simulink model "atrias_system"  (R2015a)
settings: Solver=FixedStepDiscrete  StartTime=0.0  StopTime=inf  FixedStep=sample_time  RelTol=1e-3
undefined symbols (not defined in the file or in its folder): gui_disable_cmd, gui_enable_cmd, gui_estop_cmd, gui_reset_cmd, HIP_CURRENT_LIMIT, HIP_MOTOR_CONSTANT, HIP_MTR_GEAR_RATIO, HIP_MTR_MAX_TORQUE, LEFT_MOTOR_HIP_DIRECTION, LEG1_MOTOR_A_DIRECTION, LEG1_MOTOR_B_DIRECTION, LEG2_MOTOR_A_DIRECTION, LEG2_MOTOR_B_DIRECTION, LEG_CURRENT_LIMIT, LEG_MOTOR_CONSTANT, LEG_MTR_GEAR_RATIO, LEG_MTR_MAX_TORQUE, MEDULLA_ADC_MAX_VOLTS, MEDULLA_ADC_OFFSET_COUNTS, MEDULLA_STATE_ERROR, MEDULLA_STATE_HALT, MEDULLA_STATE_IDLE, MEDULLA_STATE_RESET, MEDULLA_STATE_RUN, MOTOR_POSITION_LIMITS_LOWER, MOTOR_POSITION_LIMITS_UPPER, MTR_HIP_MAX_CURRENT, MTR_MAX_CONT_CURRENT, MTR_MAX_COUNT, MTR_MAX_CURRENT, RIGHT_MOTOR_HIP_DIRECTION
libraries: xpcethercatlib x188, simulink x36, slrtlib x2
(part 3 of 3)

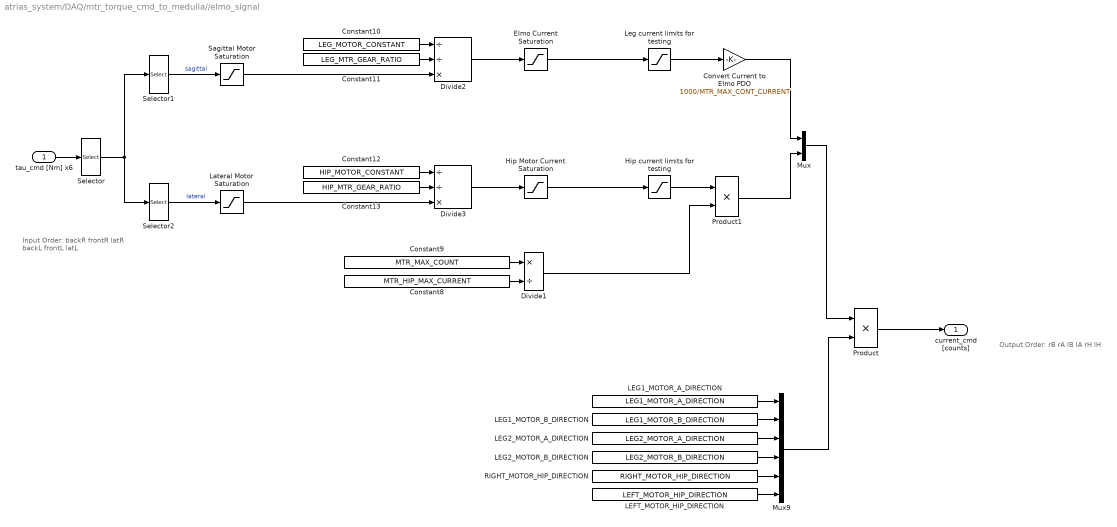
== system atrias_system/DAQ/mtr_torque_cmd_to_medulla//elmo_signal ==
  note: Output Order:
      | rB
      | rA
      | lB
      | lA
      | rH
      | lH
  note: Input Order:
      |
      | backR
      | frontR
      | latR
      | backL
      | frontL
      | latL
  tau_cmd [Nm] x6 : Inport
  Constant10 : Constant  Value=LEG_MOTOR_CONSTANT
  Constant11 : Constant  Value=LEG_MTR_GEAR_RATIO
  Constant12 : Constant  Value=HIP_MOTOR_CONSTANT
  Constant13 : Constant  Value=HIP_MTR_GEAR_RATIO
  Constant8 : Constant  Value=MTR_HIP_MAX_CURRENT
  Constant9 : Constant  Value=MTR_MAX_COUNT
  Convert Current to Elmo PDO : Gain  Gain=1000/MTR_MAX_CONT_CURRENT
  Divide1 : Product  Inputs=*/
  Divide2 : Product  Inputs=//*
  Divide3 : Product  Inputs=//*
  Elmo Current Saturation : Saturate  UpperLimit=MTR_MAX_CURRENT  LowerLimit=-MTR_MAX_CURRENT
      settings: AttributesFormatString=Top: %<UpperLimit>\nBottom: %<LowerLimit>
  Hip Motor Current Saturation : Saturate  UpperLimit=MTR_HIP_MAX_CURRENT  LowerLimit=-MTR_HIP_MAX_CURRENT
      settings: AttributesFormatString=Top: %<UpperLimit>\nBottom: %<LowerLimit>
  Hip current limits for testing : Saturate  UpperLimit=HIP_CURRENT_LIMIT  LowerLimit=-HIP_CURRENT_LIMIT
      settings: AttributesFormatString=Top: %<UpperLimit>\nBottom: %<LowerLimit>
  LEFT_MOTOR_HIP_DIRECTION : Constant  Value=LEFT_MOTOR_HIP_DIRECTION
  LEG1_MOTOR_A_DIRECTION : Constant  Value=LEG1_MOTOR_A_DIRECTION
  LEG1_MOTOR_B_DIRECTION : Constant  Value=LEG1_MOTOR_B_DIRECTION
  LEG2_MOTOR_A_DIRECTION : Constant  Value=LEG2_MOTOR_A_DIRECTION
  LEG2_MOTOR_B_DIRECTION : Constant  Value=LEG2_MOTOR_B_DIRECTION
  Lateral Motor Saturation : Saturate  UpperLimit=HIP_MTR_MAX_TORQUE  LowerLimit=-HIP_MTR_MAX_TORQUE
      settings: AttributesFormatString=Top: %<UpperLimit>\nBottom: %<LowerLimit>
  Leg current limits for testing : Saturate  UpperLimit=LEG_CURRENT_LIMIT  LowerLimit=-LEG_CURRENT_LIMIT
      settings: AttributesFormatString=Top: %<UpperLimit>\nBottom: %<LowerLimit>
  Mux : Mux  Inputs=2
  Mux9 : Mux  Inputs=6
  Product : Product  RndMeth=Zero
  Product1 : Product  RndMeth=Zero
  RIGHT_MOTOR_HIP_DIRECTION : Constant  Value=RIGHT_MOTOR_HIP_DIRECTION
  Sagittal Motor Saturation : Saturate  UpperLimit=LEG_MTR_MAX_TORQUE  LowerLimit=-LEG_MTR_MAX_TORQUE
      settings: AttributesFormatString=Top: %<UpperLimit>\nBottom: %<LowerLimit>
  Selector : Selector  InputPortWidth=6  Indices=[1 2 4 5 3 6]
  Selector1 : Selector  InputPortWidth=6  Indices=[1 2 3 4]
  Selector2 : Selector  InputPortWidth=6  Indices=[5 6]
  current_cmd [counts] : Outport
  wires:
  Lateral Motor Saturation/1 -> Divide3/3
  Sagittal Motor Saturation/1 -> Divide2/3
  Convert Current to Elmo PDO/1 -> Mux/1
  Mux/1 -> Product/1
  Divide2/1 -> Elmo Current Saturation/1
  Constant12/1 -> Divide3/1
  Constant13/1 -> Divide3/2
  Constant10/1 -> Divide2/1
  Constant11/1 -> Divide2/2
  Selector2/1 -> Lateral Motor Saturation/1  "lateral"
  Selector1/1 -> Sagittal Motor Saturation/1  "sagittal"
  LEG1_MOTOR_A_DIRECTION/1 -> Mux9/1
  LEG1_MOTOR_B_DIRECTION/1 -> Mux9/2
  LEG2_MOTOR_A_DIRECTION/1 -> Mux9/3
  Mux9/1 -> Product/2
  LEG2_MOTOR_B_DIRECTION/1 -> Mux9/4
  RIGHT_MOTOR_HIP_DIRECTION/1 -> Mux9/5
  LEFT_MOTOR_HIP_DIRECTION/1 -> Mux9/6
  Product/1 -> current_cmd [counts]/1
  tau_cmd [Nm] x6/1 -> Selector/1
  Selector/1 -> Selector1/1, Selector2/1
  Hip Motor Current Saturation/1 -> Hip current limits for testing/1
  Divide3/1 -> Hip Motor Current Saturation/1
  Constant9/1 -> Divide1/1
  Constant8/1 -> Divide1/2
  Divide1/1 -> Product1/2
  Elmo Current Saturation/1 -> Leg current limits for testing/1
  Product1/1 -> Mux/2
  Hip current limits for testing/1 -> Product1/1
  Leg current limits for testing/1 -> Convert Current to Elmo PDO/1

== system atrias_system/Start Controller/Hold Start Time ==
  Time In : Inport  OutDataTypeStr=double
  Enable : EnablePort
  Time Out : Outport  OutDataTypeStr=double
  wires:
  Time In/1 -> Time Out/1

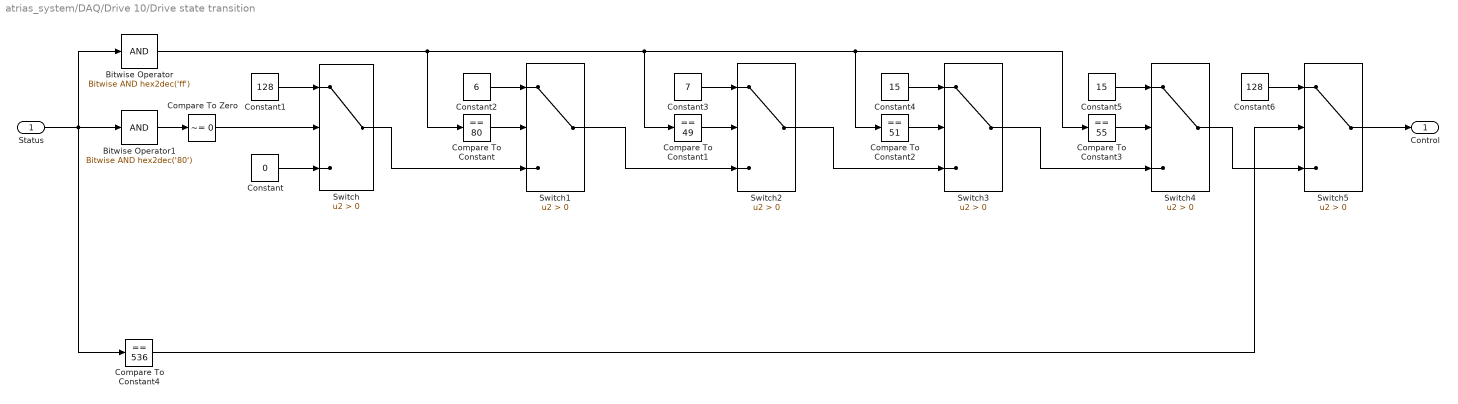
== system atrias_system/DAQ/Drive 10/Drive state transition ==
  Status : Inport
  Bitwise Operator : simulink/Logic and Bit Operations/Bitwise Operator  logicop=AND  UseBitMask=on  BitMask=hex2dec('ff')  BitMaskRealWorld=Stored Integer
  Bitwise Operator1 : simulink/Logic and Bit Operations/Bitwise Operator  logicop=AND  UseBitMask=on  BitMask=hex2dec('80')  BitMaskRealWorld=Stored Integer
  Compare To Constant : simulink/Logic and Bit Operations/Compare To Constant  relop===  const=80  OutDataTypeStr=boolean
  Compare To Constant1 : simulink/Logic and Bit Operations/Compare To Constant  relop===  const=49  OutDataTypeStr=boolean
  Compare To Constant2 : simulink/Logic and Bit Operations/Compare To Constant  relop===  const=51  OutDataTypeStr=boolean
  Compare To Constant3 : simulink/Logic and Bit Operations/Compare To Constant  relop===  const=55  OutDataTypeStr=boolean
  Compare To Constant4 : simulink/Logic and Bit Operations/Compare To Constant  relop===  const=536  OutDataTypeStr=boolean
  Compare To Zero : simulink/Logic and Bit Operations/Compare To Zero  relop=~=  OutDataTypeStr=boolean
  Constant : Constant  Value=0  OutDataTypeStr=uint16
  Constant1 : Constant  Value=128  OutDataTypeStr=uint16
  Constant2 : Constant  Value=6  OutDataTypeStr=uint16
  Constant3 : Constant  Value=7  OutDataTypeStr=uint16
  Constant4 : Constant  Value=15  OutDataTypeStr=uint16
  Constant5 : Constant  Value=15  OutDataTypeStr=uint16
  Constant6 : Constant  Value=128  OutDataTypeStr=uint16
  Switch{,1..5} (6 alike) : Switch  Criteria=u2 > Threshold
  Control : Outport
  wires:
  Constant6/1 -> Switch5/1
  Switch5/1 -> Control/1
  Compare To Constant4/1 -> Switch5/2
  Switch4/1 -> Switch5/3
  Constant5/1 -> Switch4/1
  Switch3/1 -> Switch4/3
  Compare To Constant3/1 -> Switch4/2
  Constant4/1 -> Switch3/1
  Switch2/1 -> Switch3/3
  Compare To Constant2/1 -> Switch3/2
  Constant3/1 -> Switch2/1
  Switch1/1 -> Switch2/3
  Compare To Constant1/1 -> Switch2/2
  Constant2/1 -> Switch1/1
  Bitwise Operator/1 -> Compare To Constant/1, Compare To Constant1/1, Compare To Constant2/1, Compare To Constant3/1
  Switch/1 -> Switch1/3
  Compare To Constant/1 -> Switch1/2
  Constant/1 -> Switch/3
  Constant1/1 -> Switch/1
  Compare To Zero/1 -> Switch/2
  Bitwise Operator1/1 -> Compare To Zero/1
  Status/1 -> Bitwise Operator1/1, Bitwise Operator/1, Compare To Constant4/1

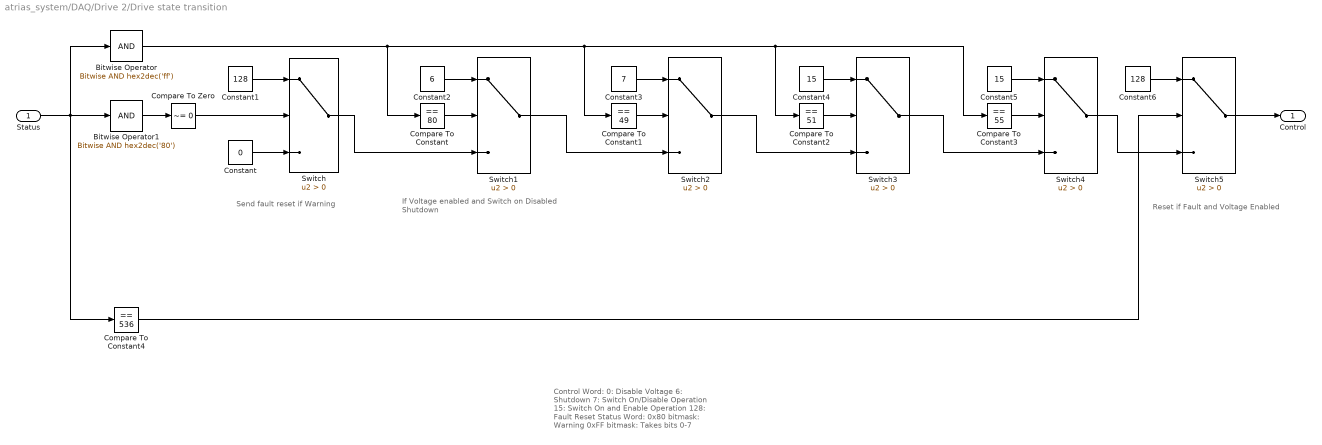
== system atrias_system/DAQ/Drive 2/Drive state transition ==
  note: If Voltage enabled and Switch on Disabled
      | Shutdown
  note: Reset if Fault and Voltage Enabled
  note: Send fault reset if Warning
  note: Control Word:
      | 0: Disable Voltage
      | 6: Shutdown
      | 7: Switch On/Disable Operation
      | 15: Switch On and Enable Operation
      | 128: Fault Reset
      |
      | Status Word:
      | 0x80 bitmask: Warning
      | 0xFF bitmask: Takes bits 0-7
  Status : Inport
  Bitwise Operator : simulink/Logic and Bit Operations/Bitwise Operator  logicop=AND  UseBitMask=on  BitMask=hex2dec('ff')  BitMaskRealWorld=Stored Integer
  Bitwise Operator1 : simulink/Logic and Bit Operations/Bitwise Operator  logicop=AND  UseBitMask=on  BitMask=hex2dec('80')  BitMaskRealWorld=Stored Integer
  Compare To Constant : simulink/Logic and Bit Operations/Compare To Constant  relop===  const=80  OutDataTypeStr=boolean
  Compare To Constant1 : simulink/Logic and Bit Operations/Compare To Constant  relop===  const=49  OutDataTypeStr=boolean
  Compare To Constant2 : simulink/Logic and Bit Operations/Compare To Constant  relop===  const=51  OutDataTypeStr=boolean
  Compare To Constant3 : simulink/Logic and Bit Operations/Compare To Constant  relop===  const=55  OutDataTypeStr=boolean
  Compare To Constant4 : simulink/Logic and Bit Operations/Compare To Constant  relop===  const=536  OutDataTypeStr=boolean
  Compare To Zero : simulink/Logic and Bit Operations/Compare To Zero  relop=~=  OutDataTypeStr=boolean
  Constant : Constant  Value=0  OutDataTypeStr=uint16
  Constant1 : Constant  Value=128  OutDataTypeStr=uint16
  Constant2 : Constant  Value=6  OutDataTypeStr=uint16
  Constant3 : Constant  Value=7  OutDataTypeStr=uint16
  Constant4 : Constant  Value=15  OutDataTypeStr=uint16
  Constant5 : Constant  Value=15  OutDataTypeStr=uint16
  Constant6 : Constant  Value=128  OutDataTypeStr=uint16
  Switch{,1..5} (6 alike) : Switch  Criteria=u2 > Threshold
  Control : Outport
  wires:
  Status/1 -> Compare To Constant4/1, Bitwise Operator/1, Bitwise Operator1/1
  Bitwise Operator1/1 -> Compare To Zero/1
  Compare To Zero/1 -> Switch/2
  Constant1/1 -> Switch/1
  Constant/1 -> Switch/3
  Compare To Constant/1 -> Switch1/2
  Switch/1 -> Switch1/3
  Bitwise Operator/1 -> Compare To Constant3/1, Compare To Constant2/1, Compare To Constant1/1, Compare To Constant/1
  Constant2/1 -> Switch1/1
  Compare To Constant1/1 -> Switch2/2
  Switch1/1 -> Switch2/3
  Constant3/1 -> Switch2/1
  Compare To Constant2/1 -> Switch3/2
  Switch2/1 -> Switch3/3
  Constant4/1 -> Switch3/1
  Compare To Constant3/1 -> Switch4/2
  Switch3/1 -> Switch4/3
  Constant5/1 -> Switch4/1
  Switch4/1 -> Switch5/3
  Compare To Constant4/1 -> Switch5/2
  Switch5/1 -> Control/1
  Constant6/1 -> Switch5/1

== system atrias_system/DAQ/Drive 3/Drive state transition ==
  Status : Inport
  Bitwise Operator : simulink/Logic and Bit Operations/Bitwise Operator  logicop=AND  UseBitMask=on  BitMask=hex2dec('ff')  BitMaskRealWorld=Stored Integer
  Bitwise Operator1 : simulink/Logic and Bit Operations/Bitwise Operator  logicop=AND  UseBitMask=on  BitMask=hex2dec('80')  BitMaskRealWorld=Stored Integer
  Compare To Constant : simulink/Logic and Bit Operations/Compare To Constant  relop===  const=80  OutDataTypeStr=boolean
  Compare To Constant1 : simulink/Logic and Bit Operations/Compare To Constant  relop===  const=49  OutDataTypeStr=boolean
  Compare To Constant2 : simulink/Logic and Bit Operations/Compare To Constant  relop===  const=51  OutDataTypeStr=boolean
  Compare To Constant3 : simulink/Logic and Bit Operations/Compare To Constant  relop===  const=55  OutDataTypeStr=boolean
  Compare To Constant4 : simulink/Logic and Bit Operations/Compare To Constant  relop===  const=536  OutDataTypeStr=boolean
  Compare To Zero : simulink/Logic and Bit Operations/Compare To Zero  relop=~=  OutDataTypeStr=boolean
  Constant : Constant  Value=0  OutDataTypeStr=uint16
  Constant1 : Constant  Value=128  OutDataTypeStr=uint16
  Constant2 : Constant  Value=6  OutDataTypeStr=uint16
  Constant3 : Constant  Value=7  OutDataTypeStr=uint16
  Constant4 : Constant  Value=15  OutDataTypeStr=uint16
  Constant5 : Constant  Value=15  OutDataTypeStr=uint16
  Constant6 : Constant  Value=128  OutDataTypeStr=uint16
  Switch{,1..5} (6 alike) : Switch  Criteria=u2 > Threshold
  Control : Outport
  wires:
  Status/1 -> Compare To Constant4/1, Bitwise Operator/1, Bitwise Operator1/1
  Bitwise Operator1/1 -> Compare To Zero/1
  Compare To Zero/1 -> Switch/2
  Constant1/1 -> Switch/1
  Constant/1 -> Switch/3
  Compare To Constant/1 -> Switch1/2
  Switch/1 -> Switch1/3
  Bitwise Operator/1 -> Compare To Constant3/1, Compare To Constant2/1, Compare To Constant1/1, Compare To Constant/1
  Constant2/1 -> Switch1/1
  Compare To Constant1/1 -> Switch2/2
  Switch1/1 -> Switch2/3
  Constant3/1 -> Switch2/1
  Compare To Constant2/1 -> Switch3/2
  Switch2/1 -> Switch3/3
  Constant4/1 -> Switch3/1
  Compare To Constant3/1 -> Switch4/2
  Switch3/1 -> Switch4/3
  Constant5/1 -> Switch4/1
  Switch4/1 -> Switch5/3
  Compare To Constant4/1 -> Switch5/2
  Switch5/1 -> Control/1
  Constant6/1 -> Switch5/1

== system atrias_system/DAQ/Drive 9/Drive state transition ==
  Status : Inport
  Bitwise Operator : simulink/Logic and Bit Operations/Bitwise Operator  logicop=AND  UseBitMask=on  BitMask=hex2dec('ff')  BitMaskRealWorld=Stored Integer
  Bitwise Operator1 : simulink/Logic and Bit Operations/Bitwise Operator  logicop=AND  UseBitMask=on  BitMask=hex2dec('80')  BitMaskRealWorld=Stored Integer
  Compare To Constant : simulink/Logic and Bit Operations/Compare To Constant  relop===  const=80  OutDataTypeStr=boolean
  Compare To Constant1 : simulink/Logic and Bit Operations/Compare To Constant  relop===  const=49  OutDataTypeStr=boolean
  Compare To Constant2 : simulink/Logic and Bit Operations/Compare To Constant  relop===  const=51  OutDataTypeStr=boolean
  Compare To Constant3 : simulink/Logic and Bit Operations/Compare To Constant  relop===  const=55  OutDataTypeStr=boolean
  Compare To Constant4 : simulink/Logic and Bit Operations/Compare To Constant  relop===  const=536  OutDataTypeStr=boolean
  Compare To Zero : simulink/Logic and Bit Operations/Compare To Zero  relop=~=  OutDataTypeStr=boolean
  Constant : Constant  Value=0  OutDataTypeStr=uint16
  Constant1 : Constant  Value=128  OutDataTypeStr=uint16
  Constant2 : Constant  Value=6  OutDataTypeStr=uint16
  Constant3 : Constant  Value=7  OutDataTypeStr=uint16
  Constant4 : Constant  Value=15  OutDataTypeStr=uint16
  Constant5 : Constant  Value=15  OutDataTypeStr=uint16
  Constant6 : Constant  Value=128  OutDataTypeStr=uint16
  Switch{,1..5} (6 alike) : Switch  Criteria=u2 > Threshold
  Control : Outport
  wires:
  Status/1 -> Compare To Constant4/1, Bitwise Operator/1, Bitwise Operator1/1
  Bitwise Operator1/1 -> Compare To Zero/1
  Compare To Zero/1 -> Switch/2
  Constant1/1 -> Switch/1
  Constant/1 -> Switch/3
  Compare To Constant/1 -> Switch1/2
  Switch/1 -> Switch1/3
  Bitwise Operator/1 -> Compare To Constant3/1, Compare To Constant2/1, Compare To Constant1/1, Compare To Constant/1
  Constant2/1 -> Switch1/1
  Compare To Constant1/1 -> Switch2/2
  Switch1/1 -> Switch2/3
  Constant3/1 -> Switch2/1
  Compare To Constant2/1 -> Switch3/2
  Switch2/1 -> Switch3/3
  Constant4/1 -> Switch3/1
  Compare To Constant3/1 -> Switch4/2
  Switch3/1 -> Switch4/3
  Constant5/1 -> Switch4/1
  Switch4/1 -> Switch5/3
  Compare To Constant4/1 -> Switch5/2
  Switch5/1 -> Control/1
  Constant6/1 -> Switch5/1

== matlab function atrias_system/DAQ/logic_voltage_volts ==
  data: u input; volt output; MEDULLA_ADC_OFFSET_COUNTS parameter; MEDULLA_ADC_MAX_VOLTS parameter
function volt = fcn(u, MEDULLA_ADC_OFFSET_COUNTS, MEDULLA_ADC_MAX_VOLTS)
% Taken from Medulla.cpp in the ATRIAS medulla drivers
% at code.google.com/p/atrias
adcReadingVolts = (u - MEDULLA_ADC_OFFSET_COUNTS) * MEDULLA_ADC_MAX_VOLTS/4095;
volt            = 6 * adcReadingVolts;

== matlab function atrias_system/DAQ/medulla_errors ==
  data: u input; errors output
function errors = fcn(u)
% right back, right front, left back, left front, left lateral, right lateral, boom
errors = reshape(bsxfun(@bitand,u,2.^[0 1 2 3 4 5 6 7]),[],1);

== matlab function atrias_system/Compute State Command ==
  data: medulla_states input uint8; elmo_enable output; medulla_cmd output; should_estop input boolean; should_halt input boolean; gui_enable_cmd parameter boolean; gui_disable_cmd parameter boolean; gui_reset_cmd parameter boolean; gui_estop_cmd parameter boolean; MEDULLA_STATE_IDLE parameter uint8; MEDULLA_STATE_RUN parameter uint8; MEDULLA_STATE_HALT parameter uint8; MEDULLA_STATE_ERROR parameter uint8; MEDULLA_STATE_RESET parameter uint8; any_halt output boolean
function [elmo_enable,medulla_cmd,any_halt] = fcn(medulla_states,      ...
                                                  should_estop,        ...
                                                  should_halt,         ...
                                                  gui_enable_cmd,      ...
                                                  gui_disable_cmd,     ...
                                                  gui_reset_cmd,       ...
                                                  gui_estop_cmd,       ...
                                                  MEDULLA_STATE_IDLE,  ...
                                                  MEDULLA_STATE_RUN,   ...
                                                  MEDULLA_STATE_HALT,  ...
                                                  MEDULLA_STATE_ERROR, ...
                                                  MEDULLA_STATE_RESET)
%#codegen

% Count the number of medullas in each state
any_idle  = any(medulla_states == MEDULLA_STATE_IDLE );
any_reset = any(medulla_states == MEDULLA_STATE_RESET);
any_run   = any(medulla_states == MEDULLA_STATE_RUN  );
any_halt  = any(medulla_states == MEDULLA_STATE_HALT );
any_estop = any(medulla_states == MEDULLA_STATE_ERROR);

% The GUI estop command should do the same thing as asserting the
% should_estop line
should_estop = should_estop || gui_estop_cmd;

% Compute whether or not to reset based on the current states and the
% GUI's input
should_reset = gui_reset_cmd  && ...
              ~gui_enable_cmd && ... % Make sure we're not about to re-enable (precaution)
               any_estop      && ... % A medulla must be e-stopped (precaution)
              ~any_halt       && ... % No medullas may be halting (precaution)
              ~any_run;              % No medullas may be running (precaution)

% Send an E-Stop first if the safeties are engaging, so this can't fail.
% Also send an E-Stop if any medullas are E-stopped, unless the GUI is
% sending a reset command
if ((any_run || any_halt) && should_estop) || (any_estop && ~should_reset)
    elmo_enable = false;
    medulla_cmd = MEDULLA_STATE_ERROR;
    return
end

% If any Medullas are halting, automatically command halt for all.
% If we want to command a halt while we're in run, command a halt.
if any_halt || (any_run && should_halt)
    elmo_enable = true;
    medulla_cmd = MEDULLA_STATE_HALT;
    return
end

% Allow for GUI-commanded resets. Make sure an enable command isn't being
% sent as an enable precaution
if should_reset || any_reset
    elmo_enable = false;
    medulla_cmd = MEDULLA_STATE_RESET;
    return
end

% Past this point, the robot should be either enabled or disabled
% (no E-Stops or halts)

% Allow the GUI to disable the robot.
% For now, there is no soft shutdown.
if gui_disable_cmd
    elmo_enable = false;
    medulla_cmd = MEDULLA_STATE_IDLE;
    return
end

% Allow for enabling (when safeties aren't triggered)
if gui_enable_cmd && ~should_estop && ~should_halt
    elmo_enable = true;
    medulla_cmd = MEDULLA_STATE_RUN;
    return
end

% Since we have no errors or relevant GUI commands, just mimic the
% Medullas's current states
if any_idle
    elmo_enable = false;
    medulla_cmd = MEDULLA_STATE_IDLE;
    return
else
    elmo_enable = true;
    medulla_cmd = MEDULLA_STATE_RUN;
    return
end
end

== matlab function atrias_system/DAQ/motor_temperatures ==
  data: u input; temp output
function temp = fcn(u)
adc_values = ((u - 172.0) * (2.70/(4095.0)));
temp = ((1.0./( (1.0/298.15) + (1.0/3988.0)*log(4700.0./((3.26./adc_values) - 1.0)/10000))) - 273.15);

== matlab function atrias_system/DAQ/motor_voltage_volts ==
  data: u input; volt output
function volt = fcn(u)
volt = (u - 1300.0) * 60.2 / (3600.0 - 1300.0);

== matlab function atrias_system/Latch Diagnostics ==
  data: reset input boolean; diags input boolean; diags_out output uint8
function diags_out = fcn(reset, diags)
%#codegen

% Recall the values of our diagnostics through a persistent variable.
% We are using a persistent variable to allow the vector to be resized
% automatically to fit the size of diags
persistent latchedDiags

% Initialize latchedDiags
if isempty(latchedDiags)
    latchedDiags = uint8(zeros(numel(diags), 1));
end


% If we're idle, then reset the counter and forward the diagnostics
% directly through.
if reset
    latchedDiags = uint8(diags);
    diags_out    = uint8(diags);
    return
end

% Since we're not idle, Sequence the diagnostics and latch the
% results    
updates    = diags & (~logical(latchedDiags));
newCounter = max(latchedDiags);
% Protect against counter overflow
if newCounter + 1 > newCounter
    newCounter = newCounter + 1;
end

% Perform the update of newly-activated diagnostic events
latchedDiags(updates) = newCounter;
diags_out             = latchedDiags;

== matlab function atrias_system/DAQ/Limit Switches to Bool ==
  data: sw input; sw_out output boolean
function sw_out  = fcn(sw)
%#codegen

% Binary decode (split the input into an array of booleans)
% This creates a matrix; each column corresponds with one of the original
% input uint8's, and each row corresponds with a bit location within the
% octet.
sw = bsxfun(@bitand, uint8(2.^(0:7)), uint8(sw(2:2:end)))';

% Reshape and cast our output to make Simulink happy
sw_out = logical(sw(:));

== matlab function atrias_system/Mux Diags ==
  data: Halting input; diags output boolean; SW input; ErrorFlags input uint8; ControllerFault input boolean; softLimits input; decelFailEstop input; transmissionLimits input
function diags = fcn(Halting, SW, ErrorFlags, ControllerFault, softLimits, decelFailEstop, transmissionLimits)
%#codegen

% Convert error flags into a boolean array.
% This will generate one column per medulla and one row per bit,
% so when we read it into diags later on it will come out in the right
% order.
ErrorFlags = logical(bsxfun(@bitand, uint8(2.^(0:7)), ErrorFlags))';

% Generate diags from the processed inputs
diags = [ Halting
          SW
          ErrorFlags(:)
          ControllerFault
          softLimits
          decelFailEstop
          transmissionLimits];

== matlab function atrias_system/Demux Diags ==
  data: diags input; halt_diag output; sw1 output; sw2 output; sw3 output; sw4 output; error1 output; error2 output; error3 output; error4 output; error5 output; error6 output; error7 output; contrlr_fault_diag output; softLimits output; decelFailEstop output; transmissionLimits output
function [halt_diag,sw1,sw2,sw3,sw4,error1,error2,error3,error4,error5,error6,error7,contrlr_fault_diag,softLimits,decelFailEstop,transmissionLimits] = fcn(diags)
%#codegen

halt_diag          = diags(1);
sw1                = diags(2:9);
sw2                = diags(10:17);
sw3                = diags(18:25);
sw4                = diags(26:33);
error1             = diags(34:41);
error2             = diags(42:49);
error3             = diags(50:57);
error4             = diags(58:65);
error5             = diags(66:73);
error6             = diags(74:81);
error7             = diags(82:89);
contrlr_fault_diag = diags(90);
softLimits         = diags(91:102);
decelFailEstop     = diags(103);
transmissionLimits = diags(104:111);

== matlab function atrias_system/Soft Limits ==
  data: estop output; q input; rotorPos input; rotorVel input; runCommand input; halt output; MOTOR_POSITION_LIMITS_UPPER parameter double; MOTOR_POSITION_LIMITS_LOWER parameter double; motorLimits output; transmissionLimits output
function [estop,halt,motorLimits,transmissionLimits] = fcn(q, ...
                                  rotorPos, ...
                                  rotorVel, ...
                                  runCommand, ...
                                  MOTOR_POSITION_LIMITS_UPPER, ...
                                  MOTOR_POSITION_LIMITS_LOWER)


%% Check the deflection between the incremental and absolute positions
% q: rBl rBm rAl rAm lBl lBm lAl lAm rHm lHm bR bY bP
% rotor: rBr rAr lBr lAr rHr lHr
% Sanity check absolute angles w.r.t. incremental angles
transmissionDfl = rotorPos(1:4)' - q([2 4 6 8]);

transmissionLimits = [transmissionDfl > 0.1
                      transmissionDfl < -0.1];

% Estop if any sensors are reporting weird data
estop = any(transmissionLimits);

% Handle encoder spikes
persistent count;
if isempty(count); count = 0; end
% If in run
if runCommand == true
    % If estop is thrown and there haven't been many bad cycles
    if estop && (count < 10)
        % Ignore the transmission limits
        estop = false;
        transmissionLimits = transmissionLimits & false;
        % Increment the count
        count = count + 1;
    end
    % If count is non-zero but estop has not been thrown
    if ~estop && (count ~= 0)
        % Reset the count
        count = 0;
    end
else % If not in run
    % Reset the counter
    count = 0;
end % if runCommand

%% Predicted stopping location at max deceleration [rad]
%    Current position + average velocity * speed   / deceleration rate
%    [rad]            + [rad/s]          * [rad/s] / ([rad/s^2/A] * [A])
rb = rotorPos(1) + rotorVel(1)/2 * abs(rotorVel(1)) / (1.7185879 * 100.0);
ra = rotorPos(2) + rotorVel(2)/2 * abs(rotorVel(2)) / (1.7185879 * 100.0);
lb = rotorPos(3) + rotorVel(3)/2 * abs(rotorVel(3)) / (1.7185879 * 100.0);
la = rotorPos(4) + rotorVel(4)/2 * abs(rotorVel(4)) / (1.7185879 * 100.0);

% Leg extension/retraction
rd = rb - ra;
ld = lb - la;

r = [ra; rb; rd];
l = [la; lb; ld];

% Check if any predicted angles are outside the safety limits
motorLimits = [r > MOTOR_POSITION_LIMITS_UPPER
               r < MOTOR_POSITION_LIMITS_LOWER
               l > MOTOR_POSITION_LIMITS_UPPER
               l < MOTOR_POSITION_LIMITS_LOWER];

halt = any(motorLimits);

end % function fcn

== matlab function atrias_system/Active Damping Safety ==
  data: tau input; tau_out output; rotorDQ input; isHalting input; decelFailEstop output
function [tau_out,decelFailEstop] = fcn(tau,rotorDQ,isHalting)

% rotor: rBr rAr lBr lAr rHr lHr
% torque: rB rA rH lB lA lH

% Deceleration initialization
persistent rB rA lB lA;
if isempty(rB)
    % Set the minimum allowable rotor velocity
    vMin = 0.3;
    rB = DampingCheck(vMin);
    rA = DampingCheck(vMin);
    lB = DampingCheck(vMin);
    lA = DampingCheck(vMin);
    % Set the current velocity as the initial velocity
    rB.initialVelocity(rotorDQ(1));
    rA.initialVelocity(rotorDQ(2));
    lB.initialVelocity(rotorDQ(3));
    lA.initialVelocity(rotorDQ(4));
end

% If everything is fine, act as a passthrough
if isHalting == false
    tau_out = tau;
    decelFailEstop = false;
    % Set the current velocity as the initial velocity
    rB.initialVelocity(rotorDQ(1));
    rA.initialVelocity(rotorDQ(2));
    lB.initialVelocity(rotorDQ(3));
    lA.initialVelocity(rotorDQ(4));
    return
end

% Damp if halting
kdlr = 600; % kd leg rotor
kdhr = 50;  % kd hip rotor
tau_out = (0 - rotorDQ([1 2 5 3 4 6])').*[kdlr kdlr kdhr kdlr kdlr kdhr]';

% E-stop if the robot fails to decelerate
decelFailTemp = [rB.checkDeceleration(rotorDQ(1))
                  rA.checkDeceleration(rotorDQ(2))
                  lB.checkDeceleration(rotorDQ(3))
                  lA.checkDeceleration(rotorDQ(4))];
decelFailEstop = any(decelFailTemp);
end % fcn
